simulink model "Get_RE_"  (R2013a)
settings: Solver=FixedStepDiscrete  StartTime=0.0  StopTime=60  RelTol=1e-3
undefined symbols (not defined in the file): ts
libraries: arduino_io_lib x12
settings Model: Creator=cell  LastModifiedBy=cell
settings OptimizationCC: OptimizeModelRefInitCode=on  LifeSpan=1
settings DebuggingCC: StrictBusMsg=Warning
settings HardwareCC: ProdBitPerInt=16  ProdBitPerPointer=8  ProdIntDivRoundTo=Zero  ProdEndianess=LittleEndian  ProdWordSize=8  ProdHWDeviceType=Atmel->AVR
settings RTWCC: SystemTargetFile=realtime.tlc  GenerateMakefile=off  TemplateMakefile=realtime.tmf  Description=Run on Target Hardware  RTWVerbose=off  ProcessScript=realtime_make_rtw_hook
settings CodeAppCC: IgnoreCustomStorageClasses=off
settings STFCustomTargetCC: TargetLibSuffix=.a  GenerateSampleERTMain=on  CombineOutputUpdateFcns=on  ERTCustomFileBanners=on  SupportContinuousTime=off  SupportNonInlinedSFcns=off  MATLABClassNameForMDSCustomization=Simulink.SoftwareTarget.ERTCustomization  SystemTargetFile=realtime.tlc
settings ERTTargetCC: ParMdlRefBuildCompliant=off  CompOptLevelCompliant=off  ConcurrentExecutionCompliant=off  ERTFirstTimeCompliant=off  ModelStepFunctionPrototypeControlCompliant=off  CPPClassGenCompliant=off  ERTCustomFileTemplate=realtime_file_process.tlc

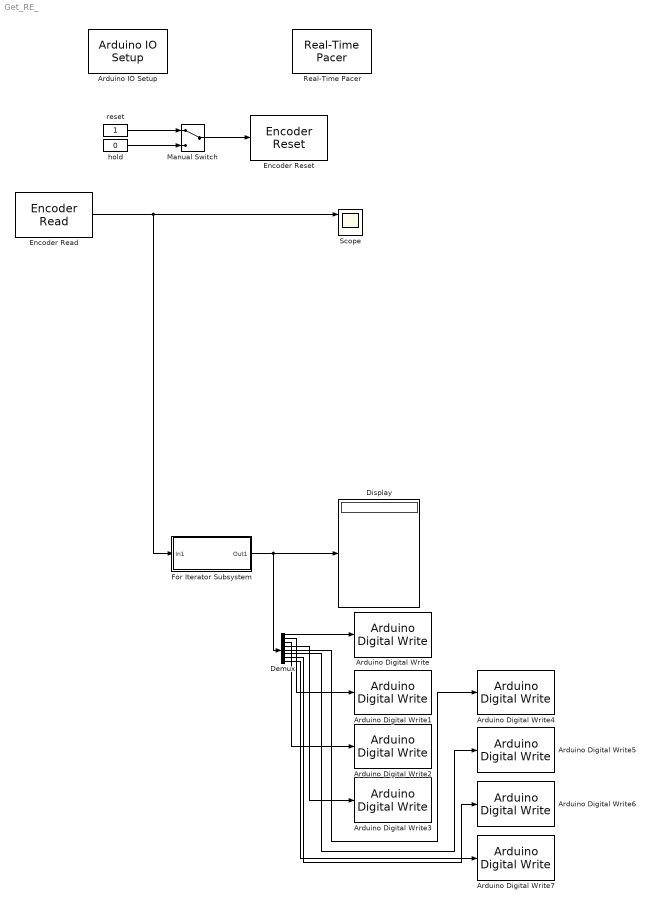
== system Get_RE_ ==
  Arduino Digital Write : arduino_io_lib/Arduino Digital Write  arduinoVar=Existing workspace arduino variable #1  arduinoPin=6  T=ts
  Arduino Digital Write1 : arduino_io_lib/Arduino Digital Write  arduinoVar=Existing workspace arduino variable #1  arduinoPin=7  T=ts
  Arduino Digital Write2 : arduino_io_lib/Arduino Digital Write  arduinoVar=Existing workspace arduino variable #1  arduinoPin=8  T=ts
  Arduino Digital Write3 : arduino_io_lib/Arduino Digital Write  arduinoVar=Existing workspace arduino variable #1  arduinoPin=9  T=ts
  Arduino Digital Write4 : arduino_io_lib/Arduino Digital Write  arduinoVar=Existing workspace arduino variable #1  arduinoPin=10  T=ts
  Arduino Digital Write5 : arduino_io_lib/Arduino Digital Write  arduinoVar=Existing workspace arduino variable #1  arduinoPin=11  T=ts
  Arduino Digital Write6 : arduino_io_lib/Arduino Digital Write  arduinoVar=Existing workspace arduino variable #1  arduinoPin=12  T=ts
  Arduino Digital Write7 : arduino_io_lib/Arduino Digital Write  arduinoVar=Existing workspace arduino variable #1  arduinoPin=13  T=ts
  Arduino IO Setup : arduino_io_lib/Arduino IO Setup  Priority=3  arduinoVar=Existing workspace arduino variable #1  workspaceVarName=a  comPort=DEMO
  Demux : Demux  Outputs=8
  Display : Display
  Encoder Read : arduino_io_lib/Encoder Read  arduinoVar=Existing workspace arduino variable #1  encNum=1  pinA=2  pinB=3  DbDl=0  T=ts
  Encoder Reset : arduino_io_lib/Encoder Reset  arduinoVar=Existing workspace arduino variable #1  encNum=1  T=ts
  For Iterator Subsystem : Subsystem  TreatAsAtomicUnit=on  mask{bits=8}
      mask prompts: bits "ビット数"
      mask Display: disp('Integer To Bit\nConvertor')
  Manual Switch : ManualSwitch
  Real-Time Pacer : arduino_io_lib/Real-Time Pacer  simTimePerRealTime=1
  Scope : Scope  NumInputPorts=3
      settings: TimeRange=10  YMin=-200~-100~0  YMax=700~100~3.75
  hold : Constant  Value=0
  reset : Constant
  wires:
  reset/1 -> Manual Switch/1
  hold/1 -> Manual Switch/2
  Manual Switch/1 -> Encoder Reset/1
  Encoder Read/1 -> For Iterator Subsystem/1(In1), Scope/1
  For Iterator Subsystem/1(Out1) -> Demux/1, Display/1
  Demux/1 -> Arduino Digital Write/1
  Demux/2 -> Arduino Digital Write1/1
  Demux/3 -> Arduino Digital Write2/1
  Demux/4 -> Arduino Digital Write3/1
  Demux/5 -> Arduino Digital Write4/1
  Demux/6 -> Arduino Digital Write5/1
  Demux/7 -> Arduino Digital Write6/1
  Demux/8 -> Arduino Digital Write7/1

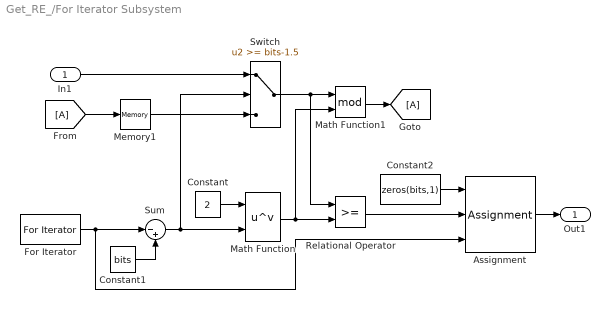
== system Get_RE_/For Iterator Subsystem ==
  In1 : Inport
  Assignment : Assignment  IndexOptions=Index vector (port)  Indices=1  OutputSizes=[1 1]
  Constant : Constant  Value=2
  Constant1 : Constant  Value=bits
  Constant2 : Constant  Value=zeros(bits,1)  VectorParams1D=off
  For Iterator : ForIterator  IterationLimit=bits
  Math Function : Math  Operator=pow  SaturateOnIntegerOverflow=on
  Math Function1 : Math  Operator=mod  SaturateOnIntegerOverflow=on
  Memory1 : Memory  InheritSampleTime=on
  Relational Operator : RelationalOperator  OutDataTypeStr=float('double')
  Sum : Sum  Inputs=|-+
  Switch : Switch  Threshold=bits-1.5
  Out1 : Outport
  wires:
  For Iterator/1 -> Sum/1, Assignment/3
  Constant/1 -> Math Function/1
  Sum/1 -> Math Function/2, Switch/2
  Constant1/1 -> Sum/2
  Math Function/1 -> Math Function1/2, Relational Operator/2
  Switch/1 -> Math Function1/1, Relational Operator/1
  In1/1 -> Switch/1
  Memory1/1 -> Switch/3
  Assignment/1 -> Out1/1
  Constant2/1 -> Assignment/1
  Relational Operator/1 -> Assignment/2
  [A] -> Memory1/1
  Math Function1/1 -> [A]
